simulink model "TaskSpaceController"  (R2024a)
settings: Solver=FixedStepDiscrete  StartTime=0.0  StopTime=Inf  FixedStep=0.001  RelTol=1e-3
model workspace (MAT data in the model file):
  robot : robotics.RigidBodyTree (value not decoded)
settings Model: Creator=sung  LastModifiedBy=sung
settings HardwareCC: ProdBitPerLong=64  ProdHWDeviceType=Intel->x86-64 (Linux 64)
settings RTWCC: GenCodeOnly=on  Toolchain=CMake

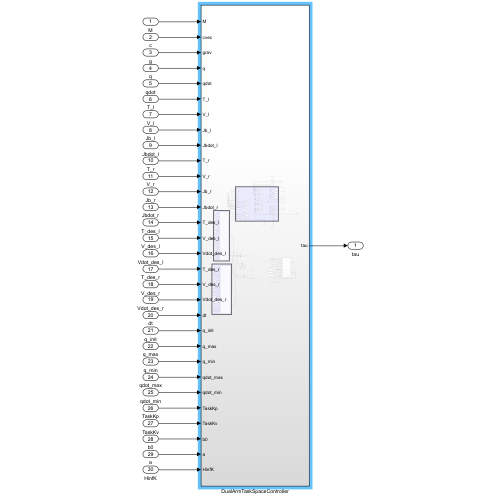
[thumbnail: Simulink's stored preview of the top-level diagram]
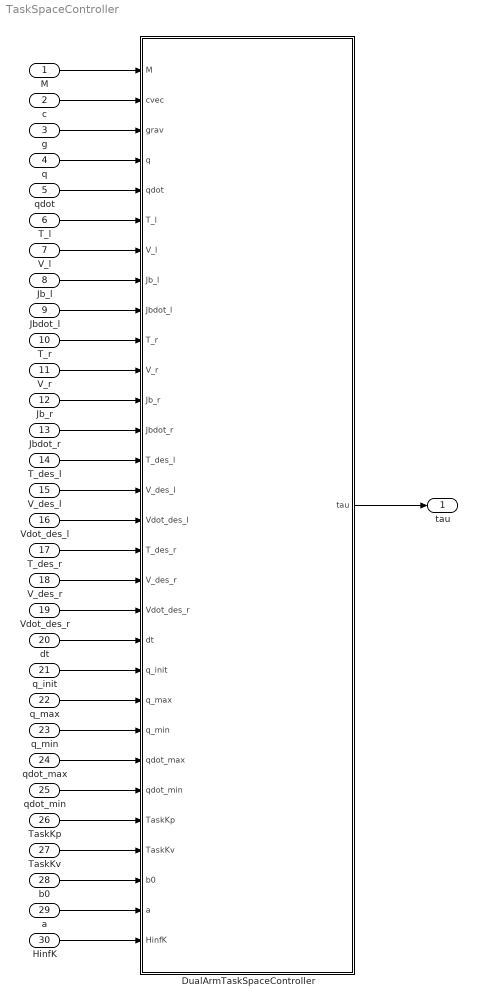
== system TaskSpaceController ==
  M : Inport  PortDimensions=[12,12]
  c : Inport  Port=2  PortDimensions=12
  g : Inport  Port=3  PortDimensions=12
  q : Inport  Port=4  PortDimensions=12
  qdot : Inport  Port=5  PortDimensions=12
  T_l : Inport  Port=6  PortDimensions=[4,4]
  V_l : Inport  Port=7  PortDimensions=6
  Jb_l : Inport  Port=8  PortDimensions=[6,6]
  Jbdot_l : Inport  Port=9  PortDimensions=[6,6]
  T_r : Inport  Port=10  PortDimensions=[4,4]
  V_r : Inport  Port=11  PortDimensions=6
  Jb_r : Inport  Port=12  PortDimensions=[6,6]
  Jbdot_r : Inport  Port=13  PortDimensions=[6,6]
  T_des_l : Inport  Port=14  PortDimensions=[4,4]
  V_des_l : Inport  Port=15  PortDimensions=6
  Vdot_des_l : Inport  Port=16  PortDimensions=6
  T_des_r : Inport  Port=17  PortDimensions=[4,4]
  V_des_r : Inport  Port=18  PortDimensions=6
  Vdot_des_r : Inport  Port=19  PortDimensions=6
  dt : Inport  Port=20
  q_init : Inport  Port=21  PortDimensions=12
  q_max : Inport  Port=22  PortDimensions=12
  q_min : Inport  Port=23  PortDimensions=12
  qdot_max : Inport  Port=24  PortDimensions=12
  qdot_min : Inport  Port=25  PortDimensions=12
  TaskKp : Inport  Port=26  PortDimensions=12
  TaskKv : Inport  Port=27  PortDimensions=12
  b0 : Inport  Port=28  PortDimensions=2
  a : Inport  Port=29  PortDimensions=2
  HinfK : Inport  Port=30  PortDimensions=12
  DualArmTaskSpaceController : Subsystem
  tau : Outport
  wires:
  qdot/1 -> DualArmTaskSpaceController/5(qdot)
  M/1 -> DualArmTaskSpaceController/1(M)
  V_r/1 -> DualArmTaskSpaceController/11(V_r)
  c/1 -> DualArmTaskSpaceController/2(cvec)
  Jb_r/1 -> DualArmTaskSpaceController/12(Jb_r)
  V_l/1 -> DualArmTaskSpaceController/7(V_l)
  g/1 -> DualArmTaskSpaceController/3(grav)
  q/1 -> DualArmTaskSpaceController/4(q)
  T_l/1 -> DualArmTaskSpaceController/6(T_l)
  Jb_l/1 -> DualArmTaskSpaceController/8(Jb_l)
  TaskKv/1 -> DualArmTaskSpaceController/27(TaskKv)
  T_des_l/1 -> DualArmTaskSpaceController/14(T_des_l)
  Jbdot_l/1 -> DualArmTaskSpaceController/9(Jbdot_l)
  T_r/1 -> DualArmTaskSpaceController/10(T_r)
  Jbdot_r/1 -> DualArmTaskSpaceController/13(Jbdot_r)
  V_des_l/1 -> DualArmTaskSpaceController/15(V_des_l)
  Vdot_des_l/1 -> DualArmTaskSpaceController/16(Vdot_des_l)
  T_des_r/1 -> DualArmTaskSpaceController/17(T_des_r)
  V_des_r/1 -> DualArmTaskSpaceController/18(V_des_r)
  q_min/1 -> DualArmTaskSpaceController/23(q_min)
  Vdot_des_r/1 -> DualArmTaskSpaceController/19(Vdot_des_r)
  dt/1 -> DualArmTaskSpaceController/20(dt)
  q_init/1 -> DualArmTaskSpaceController/21(q_init)
  q_max/1 -> DualArmTaskSpaceController/22(q_max)
  qdot_max/1 -> DualArmTaskSpaceController/24(qdot_max)
  qdot_min/1 -> DualArmTaskSpaceController/25(qdot_min)
  TaskKp/1 -> DualArmTaskSpaceController/26(TaskKp)
  b0/1 -> DualArmTaskSpaceController/28(b0)
  a/1 -> DualArmTaskSpaceController/29(a)
  HinfK/1 -> DualArmTaskSpaceController/30(HinfK)
  DualArmTaskSpaceController/1(tau) -> tau/1

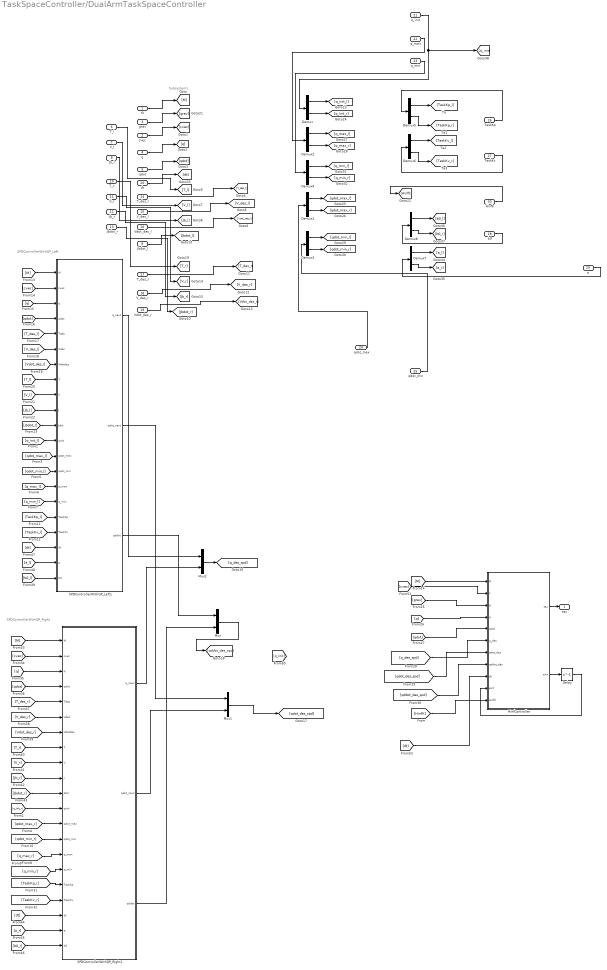
== system TaskSpaceController/DualArmTaskSpaceController ==
  note: SPDControllerWithQP_Right
  note: SPDControllerWithQP_Left
  note: Subsystem1
  M : Inport
  cvec : Inport  Port=2
  grav : Inport  Port=3
  q : Inport  Port=4
  qdot : Inport  Port=5
  T_l : Inport  Port=6
  V_l : Inport  Port=7
  Jb_l : Inport  Port=8
  Jbdot_l : Inport  Port=9
  T_r : Inport  Port=10
  V_r : Inport  Port=11
  Jb_r : Inport  Port=12
  Jbdot_r : Inport  Port=13
  T_des_l : Inport  Port=14
  V_des_l : Inport  Port=15
  Vdot_des_l : Inport  Port=16
  T_des_r : Inport  Port=17
  V_des_r : Inport  Port=18
  Vdot_des_r : Inport  Port=19
  dt : Inport  Port=20
  q_init : Inport  Port=21
  q_max : Inport  Port=22
  q_min : Inport  Port=23
  qdot_max : Inport  Port=24
  qdot_min : Inport  Port=25
  TaskKp : Inport  Port=26
  TaskKv : Inport  Port=27
  b0 : Inport  Port=28
  a : Inport  Port=29
  HinfK : Inport  Port=30
  Delay : Delay  DelayLength=1
  Demux{,1..8} (9 alike) : Demux  Outputs=2
  HinfController : MATLAB Function  TreatAsAtomicUnit=on
  Mux : Mux  Inputs=2
  Mux1 : Mux  Inputs=2
  Mux2 : Mux  Inputs=2
  SPDControllerWithQP_Left1 : MATLAB Function  TreatAsAtomicUnit=on
  SPDControllerWithQP_Right1 : MATLAB Function  TreatAsAtomicUnit=on
  tau : Outport
  wires:
  Demux/1 -> [q_init_l]
  Demux1/2 -> [qdot_max_r]
  Demux1/1 -> [qdot_max_l]
  Demux7/2 -> [a_r]
  Demux2/1 -> [q_max_l]
  Demux7/1 -> [a_l]
  qdot_max/1 -> Demux1/1
  Demux2/2 -> [q_max_r]
  V_des_r/1 -> [V_des_r]
  T_des_r/1 -> [T_des_r]
  TaskKp/1 -> Demux5/1
  qdot/1 -> [qdot]
  HinfK/1 -> [HinfK]
  T_des_l/1 -> [T_des_l]
  T_l/1 -> [T_l]
  Demux4/1 -> [q_min_l]
  Demux4/2 -> [q_min_r]
  Jbdot_r/1 -> [Jbdot_r]
  T_r/1 -> [T_r]
  Demux8/1 -> [b0_l]
  Demux8/2 -> [b0_r]
  Vdot_des_r/1 -> [Vdot_des_r]
  V_r/1 -> [V_r]
  Demux/2 -> [q_init_r]
  qdot_min/1 -> Demux3/1
  V_des_l/1 -> [V_des_l]
  Demux5/2 -> [TaskKp_r]
  Demux6/2 -> [TaskKv_r]
  Demux6/1 -> [TaskKv_l]
  q/1 -> [q]
  M/1 -> [M]
  Demux3/2 -> [qdot_min_r]
  Demux3/1 -> [qdot_min_l]
  Demux5/1 -> [TaskKp_l]
  TaskKv/1 -> Demux6/1
  Vdot_des_l/1 -> [Vdot_des_l]
  Jb_r/1 -> [Jb_r]
  dt/1 -> [dt]
  Jbdot_l/1 -> [Jbdot_l]
  grav/1 -> [grav]
  q_init/1 -> [q_init], Demux/1
  q_max/1 -> Demux2/1
  V_l/1 -> [V_l]
  q_min/1 -> Demux4/1
  b0/1 -> Demux8/1
  Jb_l/1 -> [Jb_l]
  cvec/1 -> [cvec]
  a/1 -> Demux7/1
  [q] -> HinfController/4(q)
  [qdot] -> HinfController/5(qdot)
  [M] -> HinfController/1(M)
  [HinfK] -> HinfController/11(HinfK)
  Mux/1 -> [qddot_des_spd]
  SPDControllerWithQP_Left1/3(qddot) -> Mux/1
  [grav] -> HinfController/3(g)
  SPDControllerWithQP_Right1/3(qddot) -> Mux/2
  [M] -> SPDControllerWithQP_Left1/1(M)
  [cvec] -> SPDControllerWithQP_Left1/2(cvec)
  [T_des_l] -> SPDControllerWithQP_Left1/5(Tdes)
  [qdot] -> SPDControllerWithQP_Left1/4(qdot)
  [V_des_l] -> SPDControllerWithQP_Left1/6(Vdes)
  [Vdot_des_l] -> SPDControllerWithQP_Left1/7(Vdotdes)
  [q_min_l] -> SPDControllerWithQP_Left1/16(q_min)
  [T_l] -> SPDControllerWithQP_Left1/8(T)
  [q_init_l] -> SPDControllerWithQP_Left1/12(qinit)
  [V_l] -> SPDControllerWithQP_Left1/9(V)
  [q] -> SPDControllerWithQP_Left1/3(q)
  [Jb_l] -> SPDControllerWithQP_Left1/10(J)
  [TaskKp_l] -> SPDControllerWithQP_Left1/17(TaskKp)
  [qdot_min_l] -> SPDControllerWithQP_Left1/14(qdot_min)
  [dt] -> SPDControllerWithQP_Left1/19(dt)
  [qdot_max_l] -> SPDControllerWithQP_Left1/13(qdot_max)
  [q_max_l] -> SPDControllerWithQP_Left1/15(q_max)
  [a_l] -> SPDControllerWithQP_Left1/20(a)
  [TaskKv_l] -> SPDControllerWithQP_Left1/18(TaskKv)
  [Jbdot_l] -> SPDControllerWithQP_Left1/11(Jdot)
  [b0_l] -> SPDControllerWithQP_Left1/21(b0)
  [M] -> SPDControllerWithQP_Right1/1(M)
  [q] -> SPDControllerWithQP_Right1/3(q)
  [qdot] -> SPDControllerWithQP_Right1/4(qdot)
  [cvec] -> SPDControllerWithQP_Right1/2(cvec)
  [b0_r] -> SPDControllerWithQP_Right1/21(b0)
  [qdot_min_r] -> SPDControllerWithQP_Right1/14(qdot_min)
  [V_r] -> SPDControllerWithQP_Right1/9(V)
  [Vdot_des_r] -> SPDControllerWithQP_Right1/7(Vdotdes)
  [q_max_r] -> SPDControllerWithQP_Right1/15(q_max)
  [q_min_r] -> SPDControllerWithQP_Right1/16(q_min)
  [T_r] -> SPDControllerWithQP_Right1/8(T)
  [T_des_r] -> SPDControllerWithQP_Right1/5(Tdes)
  [q_init_r] -> SPDControllerWithQP_Right1/12(qinit)
  [Jbdot_r] -> SPDControllerWithQP_Right1/11(Jdot)
  [Jb_r] -> SPDControllerWithQP_Right1/10(J)
  [dt] -> SPDControllerWithQP_Right1/19(dt)
  [a_r] -> SPDControllerWithQP_Right1/20(a)
  [qdot_max_r] -> SPDControllerWithQP_Right1/13(qdot_max)
  [V_des_r] -> SPDControllerWithQP_Right1/6(Vdes)
  [TaskKv_r] -> SPDControllerWithQP_Right1/18(TaskKv)
  [TaskKp_r] -> SPDControllerWithQP_Right1/17(TaskKp)
  HinfController/2(eint) -> Delay/1
  Delay/1 -> HinfController/10("eint ")
  HinfController/1(tau) -> tau/1
  [qddot_des_spd] -> HinfController/8(qddot_des)
  [qdot_des_spd] -> HinfController/7(qdot_des)
  [q_des_spd] -> HinfController/6(q_des)
  [cvec] -> HinfController/2(c)
  [dt] -> HinfController/9(dt)
  SPDControllerWithQP_Right1/2(qdot_next) -> Mux1/2
  SPDControllerWithQP_Left1/2(qdot_next) -> Mux1/1
  SPDControllerWithQP_Left1/1(q_next) -> Mux2/1
  SPDControllerWithQP_Right1/1(q_next) -> Mux2/2
  Mux2/1 -> [q_des_spd]
  Mux1/1 -> [qdot_des_spd]

== matlab function TaskSpaceController/DualArmTaskSpaceController/HinfController ==
  data: M input size=[12,12]; tau output size=[12,1]; c input size=[12,1]; g input size=[12,1]; q input size=[12,1]; qdot input size=[12,1]; q_des input size=[12,1]; qdot_des input size=[12,1]; qddot_des input size=[12,1]; dt input; eint input size=[12,1]; eint output; HinfK input size=[12,1]
function [tau,eint] = HinfController(M,c,g,q,qdot,q_des,qdot_des,qddot_des,dt,eint,HinfK)

e = q_des-q;
edot = qdot_des-qdot;
eint = eint+e.*dt;
qddot_ref =qddot_des+100*e+20*edot;

tau = M*qddot_ref+c+g+diag(HinfK)*(edot+20*e+100*eint);

== matlab function TaskSpaceController/DualArmTaskSpaceController/SPDControllerWithQP_Left1 ==
  data: q_next output size=[6,1]; qdot_next output size=[6,1]; M input; cvec input; q input size=[12,1]; qddot output size=[6,1]; qdot input size=[12,1]; Tdes input size=[4,4]; Vdes input size=[6,1]; Vdotdes input size=[6,1]; T input size=[4,4]; V input size=[6,1]; J input size=[6,6]; Jdot input size=[6,6]; qinit input size=[6,1]; qdot_max input size=[6,1]; qdot_min input size=[6,1]; q_max input size=[6,1]; q_min input size=[6,1]; TaskKp input size=[1,6]; TaskKv input size=[1,6]; dt input; a input; b0 input
function [q_next,qdot_next,qddot] = SPDImplicitEuler(M,cvec,q,qdot,Tdes,Vdes,Vdotdes,T,V,J,Jdot,qinit,qdot_max,qdot_min,q_max,q_min,TaskKp,TaskKv,dt,a,b0)
    % Tdes(2,4) = Tdes(2,4)+0.3*sin(2*pi*t/5);
    M = M(1:6,1:6);
    qdot  = qdot(1:6);
    q = q(1:6);
    cvec = cvec(1:6);
    q_next = q;
    qdot_next = qdot;
    % % Tdes(3,4) = Tdes(3,4)+0.5*sin(2*pi*t/5);

    TaskKp = diag(TaskKp);
    TaskKv = diag(TaskKv);


    Ttilde = TransInv(T)*Tdes;
    lambda  = log6(Ttilde);
    Vtilde = Vdes-Adjoint(TransInv(Ttilde))*V;
    dlambda = dexp6(-lambda)*Vtilde;
    AdInvT = Adjoint(TransInv(Ttilde));
    D = dlog6(-lambda)*Vdotdes-dlog6(-lambda)*AdInvT*Jdot*qdot+dlog6(-lambda)*ad(Vtilde)*Vdes-dlog6(-lambda)*ddexp6(-lambda,-dlambda)*dlambda;
    % qddot = (M+JT*TaskKv*dt*dlog6(-lambda)*AdInvT*J)\(JT*TaskKp*(lambda)+JT*TaskKp*dt*dlambda+JT*TaskKv*dlambda+(eye(7)-pinv(J)*J)*(Kinit*(qinit-q)+Dinit*(-qdot))-B*qdot);
    
    
      
    Jlambda = -dlog6(lambda)*J;
    Vtilde = Adjoint(TransInv(Ttilde))*Vdes-V;
    lambdadot = dlog6(lambda)*Vtilde;
    lambda_next = lambda+lambdadot*dt;
    B = b0 * exp(-det(J)*det(J)/ a / a) * eye(length(q));

    JlambdaT = Jlambda';
    Gamma = dlog6(lambda_next)*Adjoint(exp6(-lambda_next))*(Vdes+dt*Vdotdes)-dlog6(lambda_next)*V-dlog6(lambda_next)*dt*Jdot*qdot;
    qddot = (M+JlambdaT*TaskKv*dt*Jlambda)\(JlambdaT*(-TaskKp*lambda_next-TaskKv*Gamma)-cvec-B*qdot);
if(sum(isnan(qddot))>1)
        qddot = zeros(6,1);
    end

    % Js_prime= JacobianSpace(Slist6,q(2:end));
    % Jsdot_prime= dJacobianSpace(Js_prime,qdot(2:end));
    % Tbase_tcp =FKinSpace(M_tcp,Slist6,q(2:end));
    % p = Tbase_tcp(1:3,4);
    % pdot = Js_prime(1:3,:)*qdot(2:end);
    % 
    % 
    % p_max = 2.5;
    % lambda = 0.1;
    % 
    H = eye(6);
    % H = H+lambda*eye(6);

    f = -2*qddot;
    % f = f-lambda*qddot_prev;
    % Ao = Js_prime(1,:)*[zeros(6,1) eye(6)];

    Au = eye(6);
    bu = 10*[qdot_max-qdot];
    bl = -10*[qdot-qdot_min];
    alpha1 = 1;
    alpha3 = 10;
    beta1 = 10;
    beta3 = 100;
    Aq =eye(6);
    bqu = [-(alpha1+alpha3)*qdot+(alpha1*alpha3)*(q_max-q)];
    bql = [-(alpha1+alpha3)*qdot-(alpha1*alpha3)*(q-q_min)];
    % bou = [-(beta1+beta3)*pdot(1)+(beta1*beta3)*(p_max-p(1))-Jsdot_prime(1,:)*qdot(2:end)];

    x0 = qddot;

    A = [Au;-Au;Aq;-Aq];
    b = [bu;-bl;bqu;-bql];
    % A = [Au;-Au;Aq;-Aq];
    % b = [bu;-bl;bqu;-bql];
    options = optimoptions('quadprog', ...
                           'Algorithm','active-set', ...
                           'Display','off');

    % 4) quadprog 호출
    [x, fval, exitflag, output, lambda] = quadprog( ...
        H, f, A, b, [], [], [], [], x0, options);
    if(exitflag>0)
        qddot =x;
    else
    q_next = q+qdot*dt;
    qdot_next= qdot+qddot*dt;
    end

== matlab function TaskSpaceController/DualArmTaskSpaceController/SPDControllerWithQP_Right1 ==
  data: q_next output size=[6,1]; qdot_next output size=[6,1]; M input; cvec input; q input size=[12,1]; qddot output size=[6,1]; qdot input size=[12,1]; Tdes input size=[4,4]; Vdes input size=[6,1]; Vdotdes input size=[6,1]; T input size=[4,4]; V input size=[6,1]; J input size=[6,6]; Jdot input size=[6,6]; qinit input size=[6,1]; qdot_max input size=[6,1]; qdot_min input size=[6,1]; q_max input size=[6,1]; q_min input size=[6,1]; TaskKp input size=[1,6]; TaskKv input size=[1,6]; dt input; a input; b0 input
function [q_next,qdot_next,qddot] = SPDImplicitEuler(M,cvec,q,qdot,Tdes,Vdes,Vdotdes,T,V,J,Jdot,qinit,qdot_max,qdot_min,q_max,q_min,TaskKp,TaskKv,dt,a,b0)
    % Tdes(2,4) = Tdes(2,4)+0.3*sin(2*pi*t/5);
    M = M(7:end,7:end);
    qdot  = qdot(7:end);
    q = q(7:end);
    q_next = q;
    cvec = cvec(7:end);
    qdot_next = qdot;

    % % Tdes(3,4) = Tdes(3,4)+0.5*sin(2*pi*t/5);

    TaskKp = diag(TaskKp);
    TaskKv = diag(TaskKv);


    Ttilde = TransInv(T)*Tdes;
    lambda  = log6(Ttilde);
    Vtilde = Vdes-Adjoint(TransInv(Ttilde))*V;
    dlambda = dexp6(-lambda)*Vtilde;
    AdInvT = Adjoint(TransInv(Ttilde));
    D = dlog6(-lambda)*Vdotdes-dlog6(-lambda)*AdInvT*Jdot*qdot+dlog6(-lambda)*ad(Vtilde)*Vdes-dlog6(-lambda)*ddexp6(-lambda,-dlambda)*dlambda;
    % qddot = (M+JT*TaskKv*dt*dlog6(-lambda)*AdInvT*J)\(JT*TaskKp*(lambda)+JT*TaskKp*dt*dlambda+JT*TaskKv*dlambda+(eye(7)-pinv(J)*J)*(Kinit*(qinit-q)+Dinit*(-qdot))-B*qdot);
    
    
      
    Jlambda = -dlog6(lambda)*J;
    Vtilde = Adjoint(TransInv(Ttilde))*Vdes-V;
    lambdadot = dlog6(lambda)*Vtilde;
    lambda_next = lambda+lambdadot*dt;
    B = b0 * exp(-det(J)*det(J)/ a / a) * eye(length(q));

    JlambdaT = Jlambda';
    Gamma = dlog6(lambda_next)*Adjoint(exp6(-lambda_next))*(Vdes+dt*Vdotdes)-dlog6(lambda_next)*V-dlog6(lambda_next)*dt*Jdot*qdot;
    qddot = (M+JlambdaT*TaskKv*dt*Jlambda)\(JlambdaT*(-TaskKp*lambda_next-TaskKv*Gamma)-cvec-B*qdot);

    if(sum(isnan(qddot))>1)
        qddot = zeros(6,1);
    end
    % Js_prime= JacobianSpace(Slist6,q(2:end));
    % Jsdot_prime= dJacobianSpace(Js_prime,qdot(2:end));
    % Tbase_tcp =FKinSpace(M_tcp,Slist6,q(2:end));
    % p = Tbase_tcp(1:3,4);
    % pdot = Js_prime(1:3,:)*qdot(2:end);
    % 
    % 
    % p_max = 2.5;
    % lambda = 0.1;
    % 
    H = eye(6);
    % H = H+lambda*eye(6);

    f = -2*qddot;
    % f = f-lambda*qddot_prev;
    % Ao = Js_prime(1,:)*[zeros(6,1) eye(6)];

    Au = eye(6);
    bu = 10*[qdot_max-qdot];
    bl = -10*[qdot-qdot_min];
    alpha1 = 1;
    alpha3 = 10;
    beta1 = 10;
    beta3 = 100;
    Aq =eye(6);
    bqu = [-(alpha1+alpha3)*qdot+(alpha1*alpha3)*(q_max-q)];
    bql = [-(alpha1+alpha3)*qdot-(alpha1*alpha3)*(q-q_min)];
    % bou = [-(beta1+beta3)*pdot(1)+(beta1*beta3)*(p_max-p(1))-Jsdot_prime(1,:)*qdot(2:end)];

    x0 = qddot;

    A = [Au;-Au;Aq;-Aq];
    b = [bu;-bl;bqu;-bql];
    % A = [Au;-Au;Aq;-Aq];
    % b = [bu;-bl;bqu;-bql];
    options = optimoptions('quadprog', ...
                           'Algorithm','active-set', ...
                           'Display','off');

    % 4) quadprog 호출
    [x, fval, exitflag, output, lambda] = quadprog( ...
        H, f, A, b, [], [], [], [], x0, options);
    if(exitflag>0)
        qddot =x;
    else
    q_next =q+ qdot*dt;
    qdot_next = qdot+qddot*dt;
    end
